simulink model "lab4"  (R2015b)
settings: Solver=VariableStepAuto  SolverMode=SingleTasking  StartTime=0.0  StopTime=600  RelTol=1e-3
values from neighbouring files (symbols this model uses):
  C_obsrv = H'    [ELEC4632_lab4.m]
  DC_gain = dcgain(ss(G_obsrv-H_obsrv*L_ndb2, H_obsrv,C_obsrv, D_obsrv,Ts))    [ELEC4632_lab4.m]
  G_obsrv = G'    [ELEC4632_lab4.m]
  H_obsrv = C'    [ELEC4632_lab4.m]
  L_ndb2 = [0 1]*inv(Wc_obsrv)*P    [ELEC4632_lab4.m]
libraries: simulink x2
settings Model: Creator=jasonchen  LastModifiedBy=jasonchen
settings DataIOCC: LimitDataPoints=off
settings DebuggingCC: AllowSymbolicDim=on  SFUnexpectedBacktrackingDiag=error  SFNoUnconditionalDefaultTransitionDiag=error
settings ModelReferenceCC: PropagateSignalLabelsOutOfModel=on
settings GRTTargetCC: TargetLangStandard=C99 (ISO)
settings ConfigComp: CovMetricSettings=dwe  CovHtmlReporting=off  CovSaveCumulativeToWorkspaceVar=off  CovSaveSingleToWorkspaceVar=off  CovModelRefEnable=Off  CovExternalEMLEnable=on

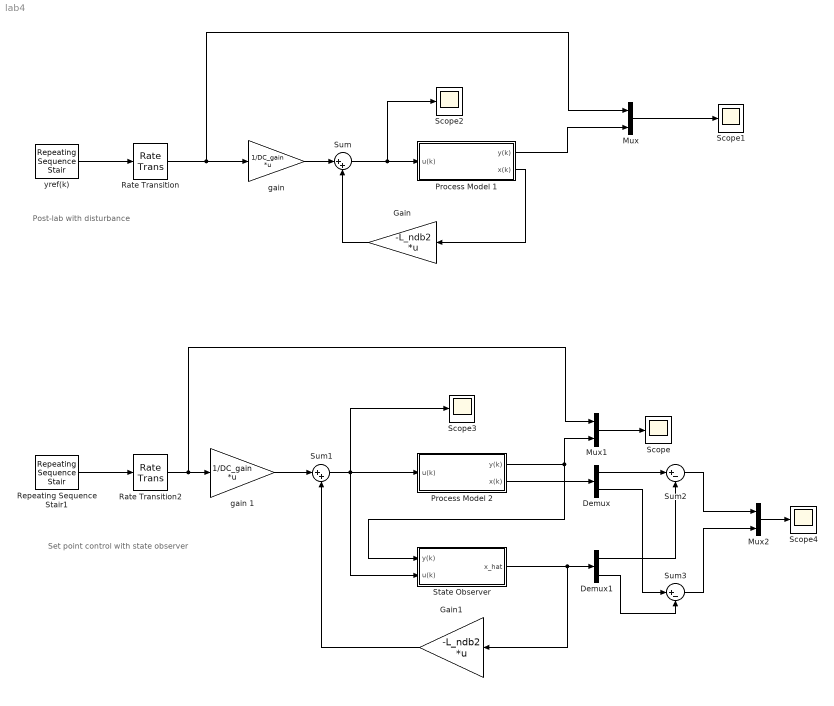
== system lab4 ==
  note: Set point control with state observer
  note: Post-lab with disturbance
  Demux : Demux  Outputs=2
  Demux1 : Demux  Outputs=2
  Gain : Gain  Gain=-L_ndb2  Multiplication=Matrix(K*u)
  Gain1 : Gain  Gain=-L_ndb2  Multiplication=Matrix(K*u)
  Mux : Mux  Inputs=2
  Mux1 : Mux  Inputs=2
  Mux2 : Mux  Inputs=2
  Process Model 1 : Subsystem
  Process Model 2 : Subsystem
  Rate Transition : RateTransition  OutPortSampleTime=0.75
  Rate Transition2 : RateTransition  OutPortSampleTime=0.75
  Repeating Sequence Stair1 : simulink/Sources/Repeating Sequence Stair  OutValues=[0 0.7 -0.2 0.5 0].'  tsamp=0.75*140  OutMin=[]  OutMax=[]  OutDataTypeStr=double  OutputDataTypeScalingMode=double  OutDataType=fixdt(0,8)  ConRadixGroup=Best Precision: Vector-wise  OutScaling=2^-12
  Scope{,1..4} (5 alike) : Scope
  "State Observer " : Subsystem
  Sum : Sum  Inputs=|++
  Sum1 : Sum  Inputs=|++
  Sum2 : Sum  Inputs=|+-
  Sum3 : Sum  Inputs=|+-
  "gain " : Gain  Gain=1/DC_gain  Multiplication=Matrix(K*u)
  gain 1 : Gain  Gain=1/DC_gain  Multiplication=Matrix(K*u)
  yref(k) : simulink/Sources/Repeating Sequence Stair  OutValues=[0 0.7 -0.2 0.5 0].'  tsamp=0.75*140  OutMin=[]  OutMax=[]  OutDataTypeStr=double  OutputDataTypeScalingMode=double  OutDataType=fixdt(0,8)  ConRadixGroup=Best Precision: Vector-wise  OutScaling=2^-12
  wires:
  Rate Transition/1 -> "gain "/1, Mux/1
  Sum/1 -> Scope2/1, Process Model 1/1(u(k))
  Process Model 1/2(x(k)) -> Gain/1
  Mux/1 -> Scope1/1
  Process Model 1/1(y(k)) -> Mux/2
  gain 1/1 -> Sum1/1
  Sum1/1 -> Scope3/1, "State Observer "/2(u(k)), Process Model 2/1(u(k))
  Process Model 2/1(y(k)) -> Mux1/2, "State Observer "/1(y(k))
  Gain1/1 -> Sum1/2
  "State Observer "/1(x_hat) -> Demux1/1, Gain1/1
  Mux1/1 -> Scope/1
  Process Model 2/2(x(k)) -> Demux/1
  Demux/1 -> Sum2/1
  Demux/2 -> Sum3/1
  Demux1/1 -> Sum2/2
  Demux1/2 -> Sum3/2
  Sum2/1 -> Mux2/1
  Sum3/1 -> Mux2/2
  Mux2/1 -> Scope4/1
  yref(k)/1 -> Rate Transition/1
  Repeating Sequence Stair1/1 -> Rate Transition2/1
  Rate Transition2/1 -> Mux1/1, gain 1/1
  "gain "/1 -> Sum/1
  Gain/1 -> Sum/2

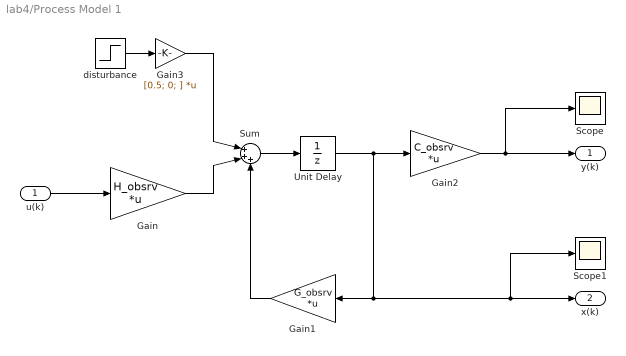
== system lab4/Process Model 1 ==
  u(k) : Inport
  Gain : Gain  Gain=H_obsrv  Multiplication=Matrix(K*u)
  Gain1 : Gain  Gain=G_obsrv  Multiplication=Matrix(K*u)
  Gain2 : Gain  Gain=C_obsrv  Multiplication=Matrix(K*u)
  Gain3 : Gain  Gain=[0.5; 0; ]  Multiplication=Matrix(K*u)
  Scope : Scope
  Scope1 : Scope
  Sum : Sum  Inputs=|+++
  Unit Delay : UnitDelay  SampleTime=0.75
  disturbance : Step  Time=100  SampleTime=0.75
  y(k) : Outport
  x(k) : Outport  Port=2
  wires:
  u(k)/1 -> Gain/1
  Sum/1 -> Unit Delay/1
  Unit Delay/1 -> Scope1/1, x(k)/1, Gain1/1, Gain2/1
  Gain2/1 -> Scope/1, y(k)/1
  disturbance/1 -> Gain3/1
  Gain1/1 -> Sum/3
  Gain/1 -> Sum/2
  Gain3/1 -> Sum/1

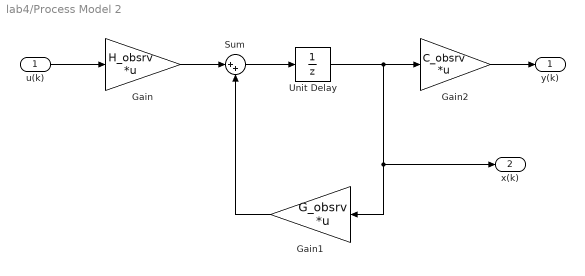
== system lab4/Process Model 2 ==
  u(k) : Inport
  Gain : Gain  Gain=H_obsrv  Multiplication=Matrix(K*u)
  Gain1 : Gain  Gain=G_obsrv  Multiplication=Matrix(K*u)
  Gain2 : Gain  Gain=C_obsrv  Multiplication=Matrix(K*u)
  Sum : Sum  Inputs=|++
  Unit Delay : UnitDelay  InitialCondition=[0;0.3]  SampleTime=0.75
  y(k) : Outport
  x(k) : Outport  Port=2
  wires:
  u(k)/1 -> Gain/1
  Sum/1 -> Unit Delay/1
  Unit Delay/1 -> Gain1/1, x(k)/1, Gain2/1
  Gain1/1 -> Sum/2
  Gain2/1 -> y(k)/1
  Gain/1 -> Sum/1

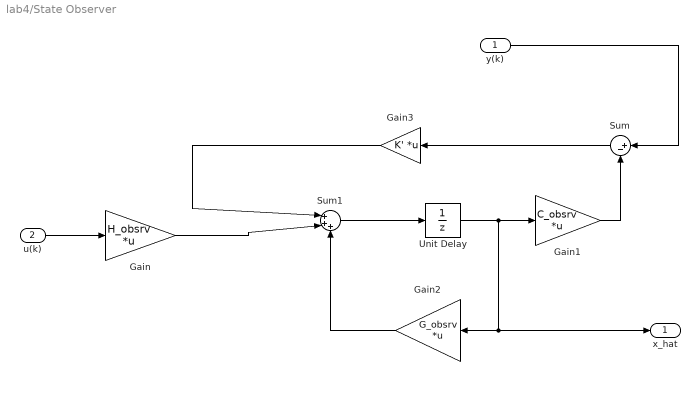
== system lab4/State Observer  ==
  y(k) : Inport
  u(k) : Inport  Port=2
  Gain : Gain  Gain=H_obsrv  Multiplication=Matrix(K*u)
  Gain1 : Gain  Gain=C_obsrv  Multiplication=Matrix(K*u)
  Gain2 : Gain  Gain=G_obsrv  Multiplication=Matrix(K*u)
  Gain3 : Gain  Gain=K'  Multiplication=Matrix(K*u)
  Sum : Sum  Inputs=|+-
  Sum1 : Sum  Inputs=|+++
  Unit Delay : UnitDelay  InitialCondition=[0;0]  SampleTime=0.75
  x_hat : Outport
  wires:
  u(k)/1 -> Gain/1
  y(k)/1 -> Sum/1
  Sum/1 -> Gain3/1
  Gain3/1 -> Sum1/1
  Gain/1 -> Sum1/2
  Sum1/1 -> Unit Delay/1
  Unit Delay/1 -> x_hat/1, Gain2/1, Gain1/1
  Gain1/1 -> Sum/2
  Gain2/1 -> Sum1/3
